simulink model "boost_converter_closed_current_voltage_loop_simscape"  (R2016a)
settings: Solver=ode23tb  StartTime=0.0  StopTime=0.2  MaxStep=0.1e-6  RelTol=1e-4
values from neighbouring files (symbols this model uses):
  C = 500e-6    (= 0.0005)    [boost_converter_current_and_voltage_loop_simscape_parameters.m]
  C2 = 1/(2*pi*R2*fzc)    [boost_converter_current_and_voltage_loop_simscape_parameters.m]
  C2v = 1/(2*pi*R2v*fzo)    [boost_converter_current_and_voltage_loop_simscape_parameters.m]
  C3 = 1/(2*pi*R2*fpc)    [boost_converter_current_and_voltage_loop_simscape_parameters.m]
  C3v = 1/(2*pi*R2v*fpo)    [boost_converter_current_and_voltage_loop_simscape_parameters.m]
  fs = 20e3    (= 20000)    [boost_converter_current_and_voltage_loop_simscape_parameters.m]
  H = 1/100    (= 0.01)    [boost_converter_current_and_voltage_loop_simscape_parameters.m]
  L = 150e-6    (= 0.00015)    [boost_converter_current_and_voltage_loop_simscape_parameters.m]
  R1 = 10e3    (= 10000)    [boost_converter_current_and_voltage_loop_simscape_parameters.m]
  R2 = Gci0*R1    [boost_converter_current_and_voltage_loop_simscape_parameters.m]
  R2v = Gcv0*R1v    [boost_converter_current_and_voltage_loop_simscape_parameters.m]
  Ra = R1v/H    (= 50000)    [boost_converter_current_and_voltage_loop_simscape_parameters.m]
  Rb = (H/(1-H))*Ra    (= 505.050505051)    [boost_converter_current_and_voltage_loop_simscape_parameters.m]
  Rload = Vo/Io    (= 16.6666666667)    [boost_converter_current_and_voltage_loop_simscape_parameters.m]
  Rs = 1    [boost_converter_current_and_voltage_loop_simscape_parameters.m]
  Vg = 200    [boost_converter_current_and_voltage_loop_simscape_parameters.m]
  VM = 1    [boost_converter_current_and_voltage_loop_simscape_parameters.m]
  Vo = 500    [boost_converter_current_and_voltage_loop_simscape_parameters.m]
libraries: powerlib x56, simulink x2
settings Model: Creator=Gorkem  LastModifiedBy=Gorkem
settings SolverCC: AlgebraicLoopSolver=LineSearch
settings GRTTargetCC: GeneratePreprocessorConditionals=Use local settings

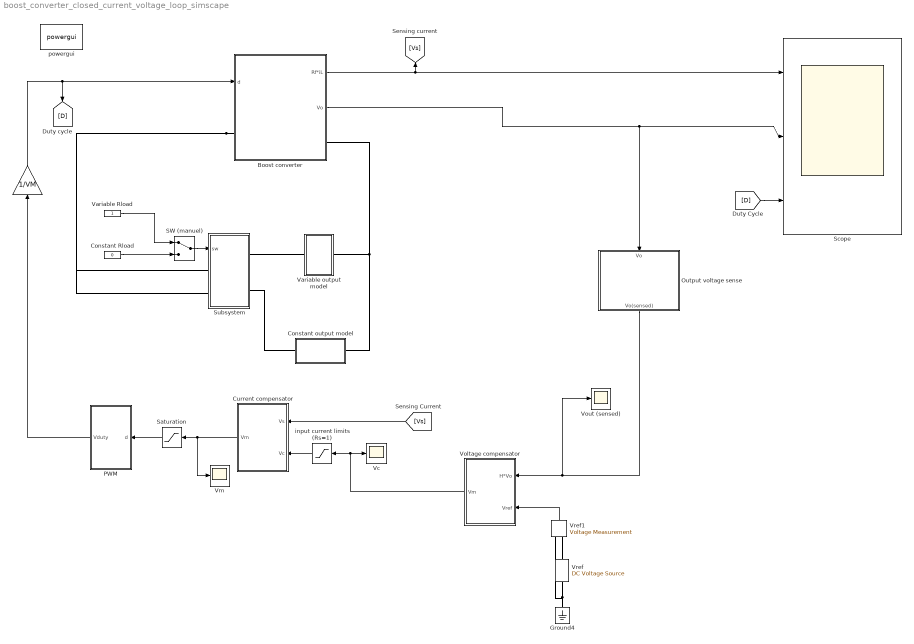
== system boost_converter_closed_current_voltage_loop_simscape ==
  "     " : Gain  Gain=1/VM
  Boost converter : Subsystem
  Constant Rload : Constant  Value=0
  Constant output model : Subsystem
  Current compensator : Subsystem
  Ground4 : powerlib/Elements/Ground  LConnTagsString=a
  Output voltage sense : Subsystem
  PWM : Subsystem
  SW (manuel) : ManualSwitch
  Saturation : Saturate  UpperLimit=1  LowerLimit=0
  Scope : Scope  NumInputPorts=3
  Subsystem : Subsystem
  Variable Rload : Constant
  Variable output model : Subsystem
  Vc : Scope
  Vm : Scope
  Voltage compensator : Subsystem
  Vout (sensed) : Scope
  Vref : powerlib/Electrical Sources/DC Voltage Source  Amplitude=H*Vo  Measurements=None
  Vref1 : powerlib/Measurements/Voltage Measurement  PhasorSimulation=off  OutputType=Complex  PSBequivalent=0
  input current limits (Rs=1) : Saturate  UpperLimit=200  LowerLimit=-200
  powergui : powerlib/powergui  Priority=1  SimulationMode=Continuous  SolverType=Tustin/Backward Euler (TBE)  SampleTime=1e-7  frequency=60  SPID=off  DisableSnubberDevices=off  DisableRonSwitches=off  DisableVfSwitches=off  SwTol=0  DisplayEquations=off  Interpol=off  ExternalGateDelay=off  methode=off  Ts=10  FunctionMessages=off  echomessages=off  HookPort=off  EnableUseOfTLC=off  x0status=blocks  frequencyindice=0  Pbase=100e6  ErrMax=1e-4  Iterations=50  UnitsV=kV  UnitsW=MW  buscounter=0  RestoreLinks=warning  ResistiveCurrentMeasurement=off  Frange=[0:2:500]  Ylog=off  Xlog=on  ShowGrid=off  save=off  variable=ZData  structure=0  ZoomFFT=off  StartTime=0.0  cycles=1  DisplayStyle=1  fundamental=60  FreqAxis=off  MaxFrequency=1000  frequencyindicesteady=1  RmsSteady=1  display=off
  wires:
  "     "/1 -> Boost converter/1(d), [D]
  Current compensator/1(Vm) -> Vm/1, Saturation/1
  PWM/1(Vduty) -> "     "/1
  input current limits (Rs=1)/1 -> Current compensator/2(Vc)
  Boost converter/1(Rf*iL) -> [Vs], Scope/1
  Boost converter/2(Vo) -> Output voltage sense/1(Vo), Scope/2
  Saturation/1 -> PWM/1(d)
  Vref1/1 -> Voltage compensator/2(Vref)
  Voltage compensator/1(Vm) -> input current limits (Rs=1)/1, Vc/1
  Variable Rload/1 -> SW (manuel)/1
  Constant Rload/1 -> SW (manuel)/2
  SW (manuel)/1 -> Subsystem/1(sw)
  Output voltage sense/1(Vo(sensed)) -> Vout (sensed)/1, Voltage compensator/1(H*Vo)
  [D] -> Scope/3
  [Vs] -> Current compensator/1(Vs)
  connections:
  Vref1/LConn1 -- Vref/RConn1
  Ground4/LConn1 -- Vref1/LConn2 -- Vref/LConn1
  Constant output model/LConn1 -- Boost converter/RConn1 -- Variable output model/RConn1
  Boost converter/LConn1 -- Subsystem/LConn2 -- Subsystem/LConn1
  Variable output model/LConn1 -- Subsystem/RConn1
  Constant output model/RConn1 -- Subsystem/RConn2

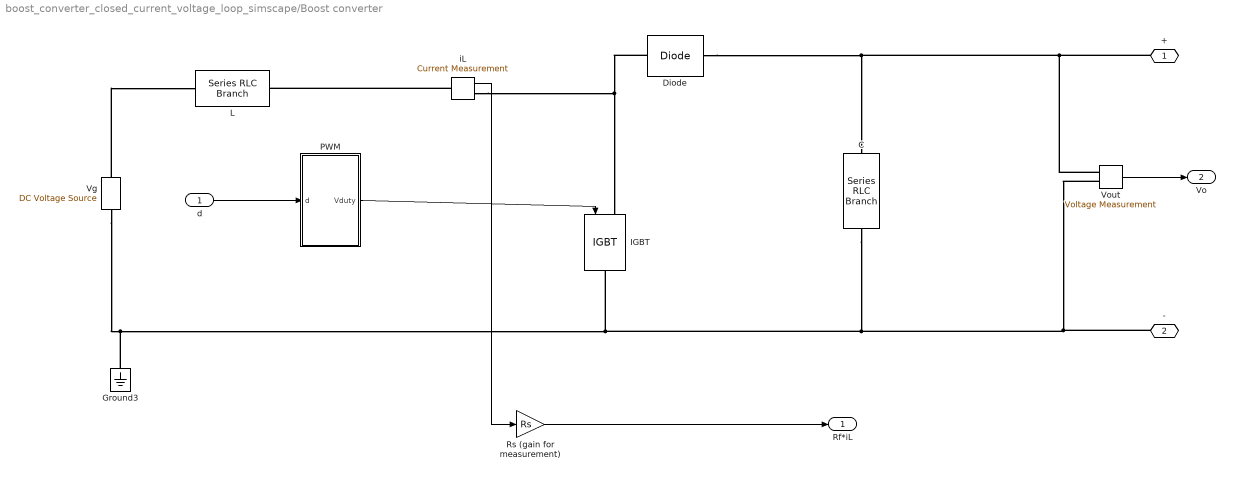
== system boost_converter_closed_current_voltage_loop_simscape/Boost converter ==
  d : Inport
  C : powerlib/Elements/Series RLC Branch  LConnTagsString=__new0  RConnTagsString=__new0  BranchType=C  Resistance=1  Inductance=L  SetiL0=off  InitialCurrent=0  Capacitance=C  Setx0=off  InitialVoltage=0  Measurements=None
  Diode : powerlib/Power Electronics/Diode  Ron=0.001  Lon=0  Vf=0.7  IC=0  UseSnubber=off  Rs=500  Cs=250e-9  Measurements=off
  Ground3 : powerlib/Elements/Ground  LConnTagsString=a
  IGBT : powerlib/Power Electronics/IGBT  Ron=0.001  Lon=0  Vf=0.7  Tf=1e-6  Tt=2e-6  IC=0  Rs=1e5  Cs=inf  Measurements=off
  L : powerlib/Elements/Series RLC Branch  LConnTagsString=__new0  RConnTagsString=__new0  BranchType=L  Resistance=1  Inductance=L  SetiL0=off  InitialCurrent=0  Capacitance=1e-6  Setx0=off  InitialVoltage=0  Measurements=None
  PWM : Subsystem
  Rs (gain for measurement) : Gain  Gain=Rs
  Vg : powerlib/Electrical Sources/DC Voltage Source  Amplitude=Vg  Measurements=None
  Vout : powerlib/Measurements/Voltage Measurement  PhasorSimulation=off  OutputType=Complex  PSBequivalent=0
  iL : powerlib/Measurements/Current Measurement  PhasorSimulation=off  OutputType=Complex  PSBequivalent=0
  + : PMIOPort  Port=1  Side=Left
  - : PMIOPort  Port=2  Side=Right
  Rf*iL : Outport
  Vo : Outport  Port=2
  wires:
  Rs (gain for measurement)/1 -> Rf*iL/1
  PWM/1(Vduty) -> IGBT/1
  d/1 -> PWM/1(d)
  iL/1 -> Rs (gain for measurement)/1
  Vout/1 -> Vo/1
  connections:
  Diode/LConn1 -- iL/RConn1 -- IGBT/LConn1
  Vout/LConn1 -- Diode/RConn1 -- C/LConn1 -- +/RConn1
  Vg/RConn1 -- L/LConn1
  iL/LConn1 -- L/RConn1
  Vg/LConn1 -- Ground3/LConn1 -- Vout/LConn2 -- -/RConn1 -- C/RConn1 -- IGBT/RConn1

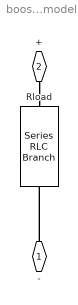
== system boost_converter_closed_current_voltage_loop_simscape/Constant output model ==
  Rload : powerlib/Elements/Series RLC Branch  LConnTagsString=__new0  RConnTagsString=__new0  BranchType=R  Resistance=Rload  Inductance=L  SetiL0=off  InitialCurrent=0  Capacitance=1e-6  Setx0=off  InitialVoltage=0  Measurements=None
  - : PMIOPort  Port=1  Side=Left
  + : PMIOPort  Port=2  Side=Right
  connections:
  -/RConn1 -- Rload/RConn1
  +/RConn1 -- Rload/LConn1

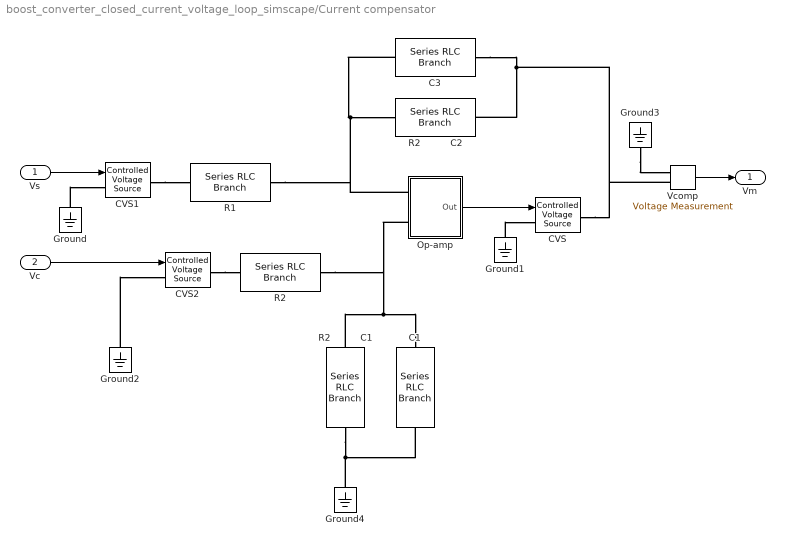
== system boost_converter_closed_current_voltage_loop_simscape/Current compensator ==
  Vs : Inport
  Vc : Inport  Port=2
  C1 : powerlib/Elements/Series RLC Branch  LConnTagsString=__new0  RConnTagsString=__new0  BranchType=C  Resistance=1  Inductance=1e-3  SetiL0=off  InitialCurrent=0  Capacitance=C3  Setx0=off  InitialVoltage=0  Measurements=None
  C3 : powerlib/Elements/Series RLC Branch  LConnTagsString=__new0  RConnTagsString=__new0  BranchType=C  Resistance=1  Inductance=1e-3  SetiL0=off  InitialCurrent=0  Capacitance=C3  Setx0=off  InitialVoltage=0  Measurements=None
  CVS : powerlib/Electrical Sources/Controlled Voltage Source  Initialize=off  Source_Type=AC  Amplitude=0  Phase=0  Frequency=0  Measurements=Voltage
  CVS1 : powerlib/Electrical Sources/Controlled Voltage Source  Initialize=off  Source_Type=DC  Amplitude=0  Phase=0  Frequency=0  Measurements=Voltage
  CVS2 : powerlib/Electrical Sources/Controlled Voltage Source  Initialize=off  Source_Type=DC  Amplitude=0  Phase=0  Frequency=0  Measurements=Voltage
  Ground{,1..4} (5 alike) : powerlib/Elements/Ground  LConnTagsString=a
  Op-amp : Subsystem
  R1 : powerlib/Elements/Series RLC Branch  LConnTagsString=__new0  RConnTagsString=__new0  BranchType=R  Resistance=R1  Inductance=1e-3  SetiL0=off  InitialCurrent=0  Capacitance=C3  Setx0=off  InitialVoltage=0  Measurements=None
  R2 : powerlib/Elements/Series RLC Branch  LConnTagsString=__new0  RConnTagsString=__new0  BranchType=R  Resistance=R1  Inductance=1e-3  SetiL0=off  InitialCurrent=0  Capacitance=C3  Setx0=off  InitialVoltage=0  Measurements=None
  R2          C1 : powerlib/Elements/Series RLC Branch  LConnTagsString=__new0  RConnTagsString=__new0  BranchType=RC  Resistance=R2  Inductance=1e-3  SetiL0=off  InitialCurrent=0  Capacitance=C2  Setx0=off  InitialVoltage=0  Measurements=None
  R2          C2 : powerlib/Elements/Series RLC Branch  LConnTagsString=__new0  RConnTagsString=__new0  BranchType=RC  Resistance=R2  Inductance=1e-3  SetiL0=off  InitialCurrent=0  Capacitance=C2  Setx0=off  InitialVoltage=0  Measurements=None
  Vcomp : powerlib/Measurements/Voltage Measurement  PhasorSimulation=off  OutputType=Complex  PSBequivalent=0
  Vm : Outport
  wires:
  Vc/1 -> CVS2/1
  Vs/1 -> CVS1/1
  Vcomp/1 -> Vm/1
  Op-amp/1(Out) -> CVS/1
  connections:
  Ground3/LConn1 -- Vcomp/LConn2
  Ground/LConn1 -- CVS1/LConn1
  CVS2/RConn1 -- R2/LConn1
  CVS1/RConn1 -- R1/LConn1
  Ground1/LConn1 -- CVS/LConn1
  Ground2/LConn1 -- CVS2/LConn1
  C3/LConn1 -- Op-amp/LConn1 -- R1/RConn1 -- R2          C2/LConn1
  C3/RConn1 -- Vcomp/LConn1 -- CVS/RConn1 -- R2          C2/RConn1
  R2          C1/RConn1 -- C1/RConn1 -- Ground4/LConn1
  R2          C1/LConn1 -- Op-amp/LConn2 -- R2/RConn1 -- C1/LConn1

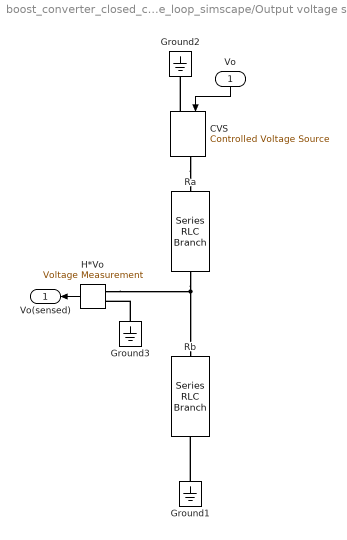
== system boost_converter_closed_current_voltage_loop_simscape/Output voltage sense ==
  Vo : Inport
  CVS : powerlib/Electrical Sources/Controlled Voltage Source  Initialize=on  Source_Type=AC  Amplitude=0  Phase=0  Frequency=0  Measurements=None
  Ground1 : powerlib/Elements/Ground  LConnTagsString=a
  Ground2 : powerlib/Elements/Ground  LConnTagsString=a
  Ground3 : powerlib/Elements/Ground  LConnTagsString=a
  H*Vo : powerlib/Measurements/Voltage Measurement  PhasorSimulation=off  OutputType=Complex  PSBequivalent=0
  Ra : powerlib/Elements/Series RLC Branch  LConnTagsString=__new0  RConnTagsString=__new0  BranchType=R  Resistance=Ra  Inductance=1e-3  SetiL0=off  InitialCurrent=0  Capacitance=C3  Setx0=off  InitialVoltage=0  Measurements=None
  Rb : powerlib/Elements/Series RLC Branch  LConnTagsString=__new0  RConnTagsString=__new0  BranchType=R  Resistance=Rb  Inductance=1e-3  SetiL0=off  InitialCurrent=0  Capacitance=C3  Setx0=off  InitialVoltage=0  Measurements=None
  Vo(sensed) : Outport
  wires:
  H*Vo/1 -> Vo(sensed)/1
  Vo/1 -> CVS/1
  connections:
  Ra/RConn1 -- Rb/LConn1 -- H*Vo/LConn1
  Ground1/LConn1 -- Rb/RConn1
  Ground3/LConn1 -- H*Vo/LConn2
  CVS/RConn1 -- Ra/LConn1
  CVS/LConn1 -- Ground2/LConn1

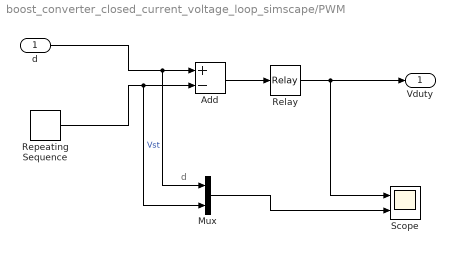
== system boost_converter_closed_current_voltage_loop_simscape/PWM ==
  note: d
  d : Inport
  Add : Sum  Inputs=+-
  Mux : Mux  Inputs=2
  Relay : Relay
  Repeating Sequence : simulink/Sources/Repeating Sequence  rep_seq_t=[0 0.001e-5 1/fs]  rep_seq_y=[1 0 1]
  Scope : Scope  NumInputPorts=2
  Vduty : Outport
  wires:
  Relay/1 -> Vduty/1, Scope/1
  Repeating Sequence/1 -> Mux/2, Add/2  "Vst"
  Add/1 -> Relay/1
  Mux/1 -> Scope/2
  d/1 -> Mux/1, Add/1

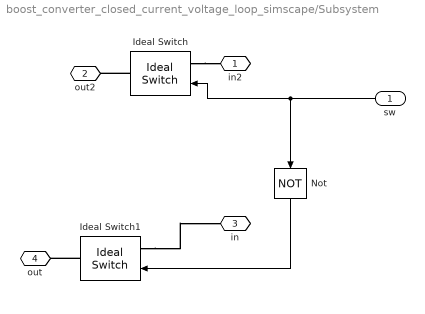
== system boost_converter_closed_current_voltage_loop_simscape/Subsystem ==
  sw : Inport
  Ideal Switch : powerlib/Power Electronics/Ideal Switch  Ron=1e-10  Lon=0  IC=0  Rs=1e5  Cs=inf  Measurements=off
  Ideal Switch1 : powerlib/Power Electronics/Ideal Switch  Ron=1e-10  Lon=0  IC=0  Rs=1e5  Cs=inf  Measurements=off
  Not : Logic  Operator=NOT  AllPortsSameDT=off  OutDataTypeStr=boolean
  in2 : PMIOPort  Port=1  Side=Right
  out2 : PMIOPort  Port=2  Side=Left
  in : PMIOPort  Port=3  Side=Right
  out : PMIOPort  Port=4  Side=Left
  wires:
  sw/1 -> Ideal Switch/1, Not/1
  Not/1 -> Ideal Switch1/1
  connections:
  Ideal Switch1/RConn1 -- out/RConn1
  Ideal Switch1/LConn1 -- in/RConn1
  Ideal Switch/LConn1 -- in2/RConn1
  Ideal Switch/RConn1 -- out2/RConn1

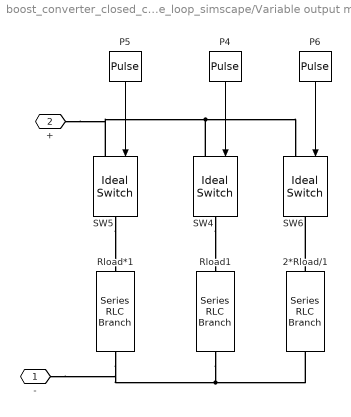
== system boost_converter_closed_current_voltage_loop_simscape/Variable output model ==
  2*Rload/1 : powerlib/Elements/Series RLC Branch  LConnTagsString=__new0  RConnTagsString=__new0  BranchType=R  Resistance=2*Rload/3  Inductance=L  SetiL0=off  InitialCurrent=0  Capacitance=1e-6  Setx0=off  InitialVoltage=0  Measurements=None
  P4 : DiscretePulseGenerator  PulseType=Time based  Period=0.2  PulseWidth=60
  P5 : DiscretePulseGenerator  PulseType=Time based  Period=0.12  PulseWidth=33  PhaseDelay=0.04
  P6 : DiscretePulseGenerator  PulseType=Time based  Period=0.2  PulseWidth=20  PhaseDelay=0.12
  Rload*1 : powerlib/Elements/Series RLC Branch  LConnTagsString=__new0  RConnTagsString=__new0  BranchType=R  Resistance=Rload  Inductance=L  SetiL0=off  InitialCurrent=0  Capacitance=1e-6  Setx0=off  InitialVoltage=0  Measurements=None
  Rload1 : powerlib/Elements/Series RLC Branch  LConnTagsString=__new0  RConnTagsString=__new0  BranchType=R  Resistance=Rload  Inductance=L  SetiL0=off  InitialCurrent=0  Capacitance=1e-6  Setx0=off  InitialVoltage=0  Measurements=None
  SW4 : powerlib/Power Electronics/Ideal Switch  Ron=1e-10  Lon=0  IC=0  Rs=1e5  Cs=inf  Measurements=off
  SW5 : powerlib/Power Electronics/Ideal Switch  Ron=1e-10  Lon=0  IC=0  Rs=1e5  Cs=inf  Measurements=off
  SW6 : powerlib/Power Electronics/Ideal Switch  Ron=1e-10  Lon=0  IC=0  Rs=1e5  Cs=inf  Measurements=off
  - : PMIOPort  Port=1  Side=Right
  + : PMIOPort  Port=2  Side=Left
  wires:
  P5/1 -> SW5/1
  P6/1 -> SW6/1
  P4/1 -> SW4/1
  connections:
  SW4/RConn1 -- Rload1/LConn1
  SW5/RConn1 -- Rload*1/LConn1
  2*Rload/1/LConn1 -- SW6/RConn1
  SW4/LConn1 -- SW5/LConn1 -- +/RConn1 -- SW6/LConn1
  Rload1/RConn1 -- 2*Rload/1/RConn1 -- Rload*1/RConn1 -- -/RConn1

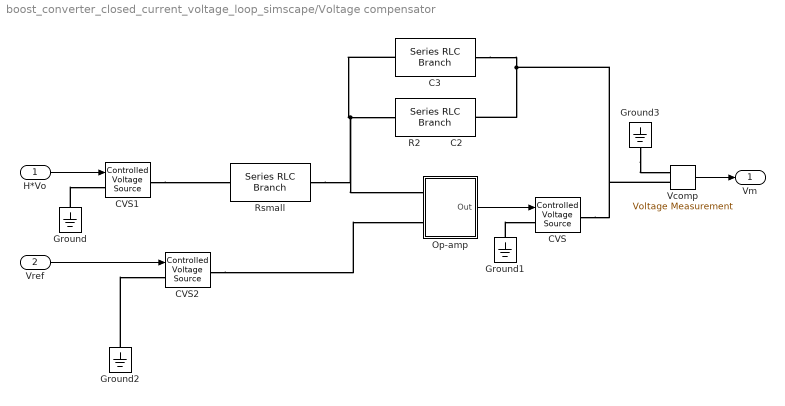
== system boost_converter_closed_current_voltage_loop_simscape/Voltage compensator ==
  H*Vo : Inport
  Vref : Inport  Port=2
  C3 : powerlib/Elements/Series RLC Branch  LConnTagsString=__new0  RConnTagsString=__new0  BranchType=C  Resistance=1  Inductance=1e-3  SetiL0=off  InitialCurrent=0  Capacitance=C3v  Setx0=off  InitialVoltage=0  Measurements=None
  CVS : powerlib/Electrical Sources/Controlled Voltage Source  Initialize=off  Source_Type=AC  Amplitude=0  Phase=0  Frequency=0  Measurements=Voltage
  CVS1 : powerlib/Electrical Sources/Controlled Voltage Source  Initialize=off  Source_Type=DC  Amplitude=0  Phase=0  Frequency=0  Measurements=Voltage
  CVS2 : powerlib/Electrical Sources/Controlled Voltage Source  Initialize=off  Source_Type=DC  Amplitude=0  Phase=0  Frequency=0  Measurements=Voltage
  Ground{,1..3} (4 alike) : powerlib/Elements/Ground  LConnTagsString=a
  Op-amp : Subsystem
  R2          C2 : powerlib/Elements/Series RLC Branch  LConnTagsString=__new0  RConnTagsString=__new0  BranchType=RC  Resistance=R2v  Inductance=1e-3  SetiL0=off  InitialCurrent=0  Capacitance=C2v  Setx0=off  InitialVoltage=0  Measurements=None
  "Rsmall " : powerlib/Elements/Series RLC Branch  LConnTagsString=__new0  RConnTagsString=__new0  BranchType=R  Resistance=Ra*Rb/(Ra+Rb)  Inductance=1e-3  SetiL0=off  InitialCurrent=0  Capacitance=C3v  Setx0=off  InitialVoltage=0  Measurements=None
  Vcomp : powerlib/Measurements/Voltage Measurement  PhasorSimulation=off  OutputType=Complex  PSBequivalent=0
  Vm : Outport
  wires:
  Vref/1 -> CVS2/1
  H*Vo/1 -> CVS1/1
  Vcomp/1 -> Vm/1
  Op-amp/1(Out) -> CVS/1
  connections:
  Ground3/LConn1 -- Vcomp/LConn2
  Ground/LConn1 -- CVS1/LConn1
  Ground1/LConn1 -- CVS/LConn1
  Ground2/LConn1 -- CVS2/LConn1
  C3/LConn1 -- Op-amp/LConn1 -- "Rsmall "/RConn1 -- R2          C2/LConn1
  C3/RConn1 -- Vcomp/LConn1 -- CVS/RConn1 -- R2          C2/RConn1
  CVS2/RConn1 -- Op-amp/LConn2
  CVS1/RConn1 -- "Rsmall "/LConn1

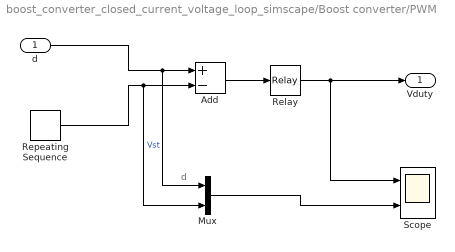
== system boost_converter_closed_current_voltage_loop_simscape/Boost converter/PWM ==
  note: d
  d : Inport
  Add : Sum  Inputs=+-
  Mux : Mux  Inputs=2
  Relay : Relay
  Repeating Sequence : simulink/Sources/Repeating Sequence  rep_seq_t=[0 1e-7 1/fs]  rep_seq_y=[1 0 1]
  Scope : Scope  NumInputPorts=2
  Vduty : Outport
  wires:
  Relay/1 -> Vduty/1, Scope/1
  Repeating Sequence/1 -> Mux/2, Add/2  "Vst"
  Add/1 -> Relay/1
  Mux/1 -> Scope/2
  d/1 -> Mux/1, Add/1

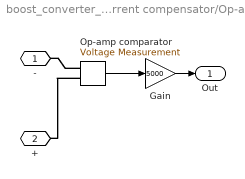
== system boost_converter_closed_current_voltage_loop_simscape/Current compensator/Op-amp ==
  Gain : Gain  Gain=5000
  "Op-amp comparator " : powerlib/Measurements/Voltage Measurement  PhasorSimulation=off  OutputType=Complex  PSBequivalent=0
  - : PMIOPort  Port=1  Side=Left
  + : PMIOPort  Port=2  Side=Left
  Out : Outport
  wires:
  Gain/1 -> Out/1
  "Op-amp comparator "/1 -> Gain/1
  connections:
  "Op-amp comparator "/LConn1 -- +/RConn1
  "Op-amp comparator "/LConn2 -- -/RConn1

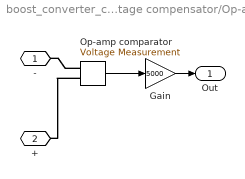
== system boost_converter_closed_current_voltage_loop_simscape/Voltage compensator/Op-amp ==
  Gain : Gain  Gain=5000
  "Op-amp comparator " : powerlib/Measurements/Voltage Measurement  PhasorSimulation=off  OutputType=Complex  PSBequivalent=0
  - : PMIOPort  Port=1  Side=Left
  + : PMIOPort  Port=2  Side=Left
  Out : Outport
  wires:
  Gain/1 -> Out/1
  "Op-amp comparator "/1 -> Gain/1
  connections:
  "Op-amp comparator "/LConn1 -- +/RConn1
  "Op-amp comparator "/LConn2 -- -/RConn1
